simulink model "State_Space_A01735217 (1)"  (R2024a)
settings: Solver=VariableStepAuto  StartTime=0.0  StopTime=100  RelTol=1e-3

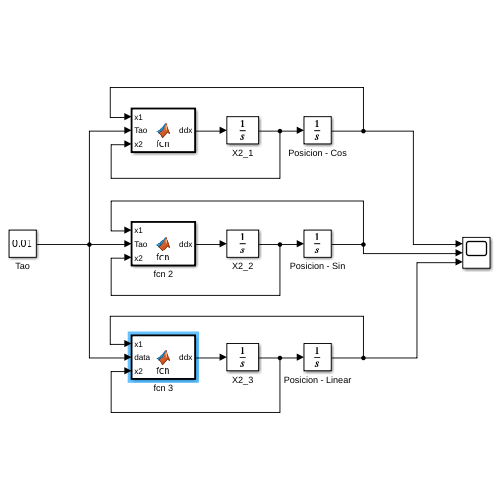
[thumbnail: Simulink's stored preview of the top-level diagram]
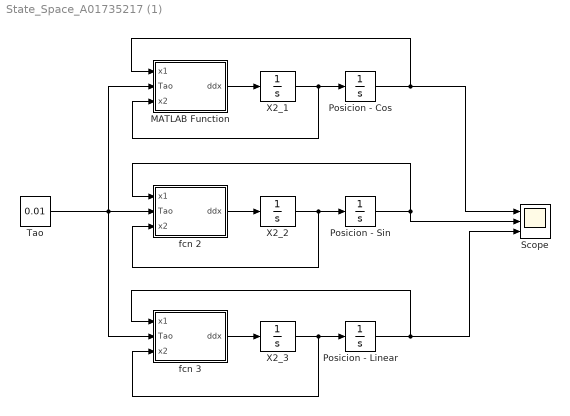
== system State_Space_A01735217 (1) ==
  MATLAB Function : MATLAB Function  TreatAsAtomicUnit=on
  Posicion - Cos : Integrator  InitialCondition=pi/20
  Posicion - Linear : Integrator  InitialCondition=pi/20
  Posicion - Sin : Integrator  InitialCondition=pi/20
  Scope : Scope  NumInputPorts=3
  Tao : Constant  Value=0.01
  X2_1 : Integrator
  X2_2 : Integrator
  X2_3 : Integrator
  fcn 2 : MATLAB Function  TreatAsAtomicUnit=on
  fcn 3 : MATLAB Function  TreatAsAtomicUnit=on
  wires:
  X2_1/1 -> MATLAB Function/3(x2), Posicion - Cos/1
  MATLAB Function/1(ddx) -> X2_1/1
  Posicion - Cos/1 -> MATLAB Function/1(x1), Scope/1
  X2_2/1 -> fcn 2/3(x2), Posicion - Sin/1
  fcn 2/1(ddx) -> X2_2/1
  Posicion - Sin/1 -> fcn 2/1(x1), Scope/2
  X2_3/1 -> fcn 3/3(x2), Posicion - Linear/1
  fcn 3/1(ddx) -> X2_3/1
  Posicion - Linear/1 -> fcn 3/1(x1), Scope/3
  Tao/1 -> fcn 3/2(Tao), MATLAB Function/2(Tao), fcn 2/2(Tao)

== matlab function State_Space_A01735217 (1)/MATLAB Function ==
  data: x1 input; Tao input; x2 input; ddx output
function ddx = fcn(x1,Tao, x2)

k = 0.01;
m = 0.75;
l = 0.36;
g = 9.8;

%Arguments calculation
a= l/2;
J = 4/3*m*a*a;

ddx=Tao/J - k*x2/J -m*g*a*cos(x1)/J;
end

== matlab function State_Space_A01735217 (1)/fcn 3 ==
  data: x1 input; Tao input; x2 input; ddx output
function ddx = fcn(x1,Tao, x2)

k = 0.01;
m = 0.75;
l = 0.36;
g = 9.8;

%Arguments calculation
a= l/2;
J = 4/3*m*a*a;

ddx=Tao/J - k*x2/J -m*g*a*x1/J;
end

== matlab function State_Space_A01735217 (1)/fcn 2 ==
  data: x1 input; Tao input; x2 input; ddx output
function ddx = fcn(x1,Tao, x2)

k = 0.01;
m = 0.75;
l = 0.36;
g = 9.8;

%Arguments calculation
a= l/2;
J = 4/3*m*a*a;

ddx=Tao/J - k*x2/J -m*g*a*sin(x1)/J;
end
